simulink library "LIB_TF_G_12_StepControl"  (Simulink 8.6)
settings: Solver=ode45  StartTime=0.0  StopTime=10.0  RelTol=1e-3
PreLoadFcn:
  | if exist('tl_preloadfcn','file'), tl_preloadfcn(gcs,402); end
PostLoadFcn:
  | if exist('tl_postloadfcn','file'), tl_postloadfcn(gcs,402); end
undefined symbols (not defined in the file): ddv, u2, u3
libraries: tllib x4, LIB_TF_G_12_StepControl x1
(part 1 of 7)
CloseFcn:
  | if exist('tl_closefcn','file'), tl_closefcn(gcs); end
settings Model: TLRevision=402  Creator=cedric.sauvage  LastModifiedBy=audrey.vache

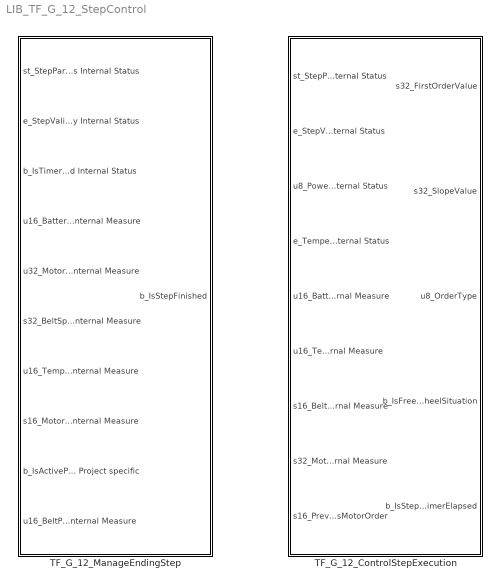
== system LIB_TF_G_12_StepControl ==
  TF_G_12_ControlStepExecution : Subsystem  TreatAsAtomicUnit=on
  TF_G_12_ManageEndingStep : Subsystem  TreatAsAtomicUnit=on

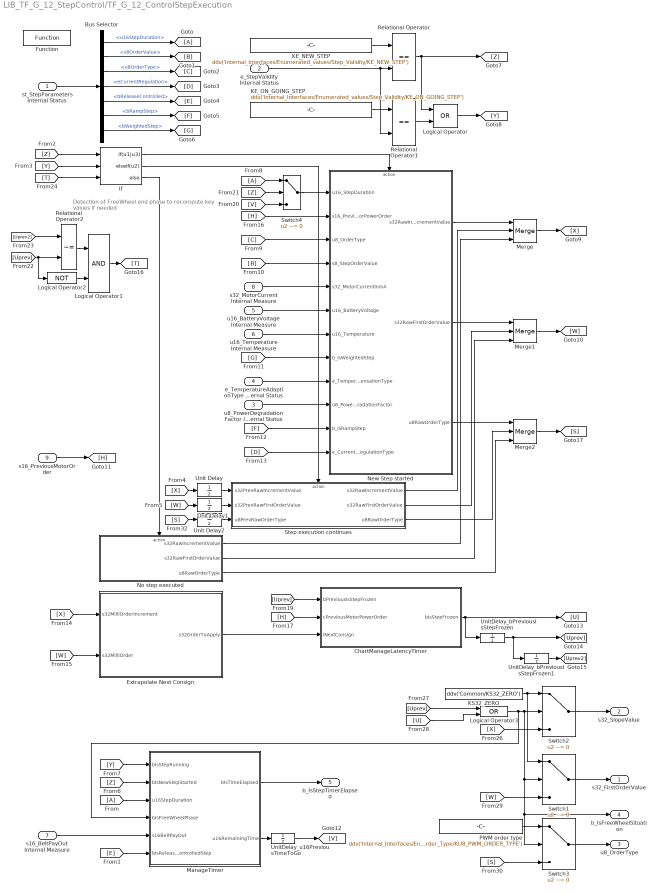
== system LIB_TF_G_12_StepControl/TF_G_12_ControlStepExecution ==
  note: Detection of FreeWheel end phase to recompute
      | key values if needed
  st_StepParameters Internal Status : Inport  OutDataTypeStr=Bus: stStepParameters
  e_StepValidity Internal Status : Inport  Port=2
  u8_PowerDegradationFactor Internal Status : Inport  Port=3
  e_TemperatureAdaptionType Internal Status : Inport  Port=4
  u16_BatteryVoltage Internal Measure : Inport  Port=5
  u16_Temperature Internal Measure : Inport  Port=6
  s16_BeltPayOut Internal Measure : Inport  Port=7
  s32_MotorCurrent Internal Measure : Inport  Port=8
  s16_PreviousMotorOrder : Inport  Port=9
  Bus Selector : BusSelector  OutputSignals=u16StepDuration,s8OrderValue,u8OrderType,eCurrentRegulation,bReleaseControlled,bRampStep,bWeightedStep
  ChartManageLatencyTimer : Stateflow chart  RequirementInfo={} %GIDa_4b5a57f6_b7b0_49a6_a1eb_944317c1d2de  TreatAsAtomicUnit=on
  Extrapolate Next Consign : Subsystem  RequirementInfo={} %GIDa_72e94147_9b66_478c_94cc_c32d89e0e2b0  TreatAsAtomicUnit=on
  Function : tllib/Function  RequirementInfo={'other' '..\..\..\..\Documents and Settings\cedric.sauvage\Desktop\BFE_Design.doc' '@Simulink_requirement_item_16' 'true' 'DSG_BFE_00033' '' } %GIDa_aa7399e7_4aec_40ce_b84e_da620cbb38ff  data={'stepfunctionname','M_ControlStepExecution','stepfunctionclass','STATIC_FCN_ASR4','codecomment',['[COVERS: DSG_BFE_00033]'],'date',736467.70154953701}  displayString=FUNCTION
  If : If  RequirementInfo={} %GIDa_dfdbd0a4_334d_4bd1_9cca_3fcb5b10a1a1  NumInputs=3  IfExpression=u1|u3  ElseIfExpressions=u2
  KE_NEW_STEP : Constant  Value=ddv('Internal_Interfaces/Enumerated_values/Step_Validity/KE_NEW_STEP')  mask(TL_Constant){data={'output',{'variable','Internal_Interfaces/Enumerated_values/Step_Validity/KE_NEW_STEP'},'date',735951.6680056944}}
      settings: CopyFcn=if exist('tl_reset_reviewflag','file')==2,tl_reset_reviewflag(gcbh);end  DeleteFcn=if exist('delete_tlblock','file')==2,delete_tlblock(gcbh);end  NameChangeFcn=if exist('rename_tlblock','file')==2,rename_tlblock(gcbh);end  OpenFcn=if exist('tl_open_blockdlg','file')==2,tl_open_blockdlg(gcbh);else,open_system(gcbh,'parameter');end
      mask Help: eval(['if exist(''tl_online_help'',''file'') == 2, tl_online_help(''Topic'',''TL_Constant''),else, web([''jar:file:///'',matlabroot,''/help/toolbox/simulink/help.jar!/slref/' lower(get_param(gcbh,'Blocktype')) '.html''], ''-helpbrowser''),end'])
      mask Display: plot([-0.05, 1.05, NaN, -0.05, 1.05],[.01, .01, NaN, .99, .99])
  KE_ON_GOING_STEP : Constant  Value=ddv('Internal_Interfaces/Enumerated_values/Step_Validity/KE_ON_GOING_STEP')  mask(TL_Constant){data={'output',{'variable','Internal_Interfaces/Enumerated_values/Step_Validity/KE_ON_GOING_STEP'},'date',735951.66800531244}}
      settings: CopyFcn=if exist('tl_reset_reviewflag','file')==2,tl_reset_reviewflag(gcbh);end  DeleteFcn=if exist('delete_tlblock','file')==2,delete_tlblock(gcbh);end  NameChangeFcn=if exist('rename_tlblock','file')==2,rename_tlblock(gcbh);end  OpenFcn=if exist('tl_open_blockdlg','file')==2,tl_open_blockdlg(gcbh);else,open_system(gcbh,'parameter');end
      mask Help: eval(['if exist(''tl_online_help'',''file'') == 2, tl_online_help(''Topic'',''TL_Constant''),else, web([''jar:file:///'',matlabroot,''/help/toolbox/simulink/help.jar!/slref/' lower(get_param(gcbh,'Blocktype')) '.html''], ''-helpbrowser''),end'])
      mask Display: plot([-0.05, 1.05, NaN, -0.05, 1.05],[.01, .01, NaN, .99, .99])
  KS32_ZERO : Constant  RequirementInfo={} %GIDa_9199cee5_bc37_4797_a880_19721e26adfa  Value=ddv('Common/KS32_ZERO')  OutDataTypeStr=int32  mask(TL_Constant){data={'output',{'variable','Common/KS32_ZERO'},'date',735951.66800494213}}
      settings: CopyFcn=if exist('tl_reset_reviewflag','file')==2,tl_reset_reviewflag(gcbh);end  DeleteFcn=if exist('delete_tlblock','file')==2,delete_tlblock(gcbh);end  NameChangeFcn=if exist('rename_tlblock','file')==2,rename_tlblock(gcbh);end  OpenFcn=if exist('tl_open_blockdlg','file')==2,tl_open_blockdlg(gcbh);else,open_system(gcbh,'parameter');end
      mask Help: eval(['if exist(''tl_online_help'',''file'') == 2, tl_online_help(''Topic'',''TL_Constant''),else, web([''jar:file:///'',matlabroot,''/help/toolbox/simulink/help.jar!/slref/' lower(get_param(gcbh,'Blocktype')) '.html''], ''-helpbrowser''),end'])
      mask Display: plot([-0.05, 1.05, NaN, -0.05, 1.05],[.01, .01, NaN, .99, .99])
  Logical Operator : Logic  Operator=OR  AllPortsSameDT=off  OutDataTypeStr=boolean  mask(TL_LogicalOperator){data={'output',{'name','bIsActiveStep'},'date',735951.66800458333}}
      settings: DeleteFcn=if exist('delete_tlblock','file')==2,delete_tlblock(gcbh);end  NameChangeFcn=if exist('rename_tlblock','file')==2,rename_tlblock(gcbh);end  OpenFcn=if exist('tl_open_blockdlg','file')==2,tl_open_blockdlg(gcbh);else,open_system(gcbh,'parameter');end
      mask Help: eval(['if exist(''tl_online_help'',''file'') == 2, tl_online_help(''Topic'',''TL_LogicalOperator''),else, web([''jar:file:///'',matlabroot,''/help/toolbox/simulink/help.jar!/slref/' lower(get_param(gcbh,'Blocktype')) '.html''], ''-helpbrowser''),end'])
      mask Display: plot([-0.05, 1.05, NaN, -0.05, 1.05],[.01, .01, NaN, .99, .99])
  Logical Operator1 : Logic  AllPortsSameDT=off  OutDataTypeStr=boolean  mask(TL_LogicalOperator){data={'output',{'name','bExitingFrozenState'},'date',735951.66800432873}}
      settings: DeleteFcn=if exist('delete_tlblock','file')==2,delete_tlblock(gcbh);end  NameChangeFcn=if exist('rename_tlblock','file')==2,rename_tlblock(gcbh);end  OpenFcn=if exist('tl_open_blockdlg','file')==2,tl_open_blockdlg(gcbh);else,open_system(gcbh,'parameter');end
      mask Help: eval(['if exist(''tl_online_help'',''file'') == 2, tl_online_help(''Topic'',''TL_LogicalOperator''),else, web([''jar:file:///'',matlabroot,''/help/toolbox/simulink/help.jar!/slref/' lower(get_param(gcbh,'Blocktype')) '.html''], ''-helpbrowser''),end'])
      mask Display: plot([-0.05, 1.05, NaN, -0.05, 1.05],[.01, .01, NaN, .99, .99])
  Logical Operator2 : Logic  Operator=NOT  Inputs=1  AllPortsSameDT=off  OutDataTypeStr=boolean  mask(TL_LogicalOperator){data={'date',735951.66800407402}}
      settings: DeleteFcn=if exist('delete_tlblock','file')==2,delete_tlblock(gcbh);end  NameChangeFcn=if exist('rename_tlblock','file')==2,rename_tlblock(gcbh);end  OpenFcn=if exist('tl_open_blockdlg','file')==2,tl_open_blockdlg(gcbh);else,open_system(gcbh,'parameter');end
      mask Help: eval(['if exist(''tl_online_help'',''file'') == 2, tl_online_help(''Topic'',''TL_LogicalOperator''),else, web([''jar:file:///'',matlabroot,''/help/toolbox/simulink/help.jar!/slref/' lower(get_param(gcbh,'Blocktype')) '.html''], ''-helpbrowser''),end'])
      mask Display: plot([-0.05, 1.05, NaN, -0.05, 1.05],[.01, .01, NaN, .99, .99])
  Logical Operator3 : Logic  Operator=OR  AllPortsSameDT=off  OutDataTypeStr=boolean  mask(TL_LogicalOperator){data={'output',{'name','bIsFreeWheelingState'},'date',735951.66800378473}}
      settings: DeleteFcn=if exist('delete_tlblock','file')==2,delete_tlblock(gcbh);end  NameChangeFcn=if exist('rename_tlblock','file')==2,rename_tlblock(gcbh);end  OpenFcn=if exist('tl_open_blockdlg','file')==2,tl_open_blockdlg(gcbh);else,open_system(gcbh,'parameter');end
      mask Help: eval(['if exist(''tl_online_help'',''file'') == 2, tl_online_help(''Topic'',''TL_LogicalOperator''),else, web([''jar:file:///'',matlabroot,''/help/toolbox/simulink/help.jar!/slref/' lower(get_param(gcbh,'Blocktype')) '.html''], ''-helpbrowser''),end'])
      mask Display: plot([-0.05, 1.05, NaN, -0.05, 1.05],[.01, .01, NaN, .99, .99])
  ManageTimer : Subsystem  RequirementInfo={} %GIDa_1c6e116c_deb6_4c8b_9c2a_a3ed8f535171  TreatAsAtomicUnit=on
      settings: RTWFcnNameOpts=Use subsystem name
  Merge : Merge  Inputs=3  InitialOutput=0  mask(TL_Merge){data={'output',{'name','s32RawIncrementValue'},'date',735951.66799646989}}
      settings: CopyFcn=if exist('tl_reset_reviewflag','file')==2,tl_reset_reviewflag(gcbh);end  DeleteFcn=if exist('delete_tlblock','file')==2,delete_tlblock(gcbh);end  NameChangeFcn=if exist('rename_tlblock','file')==2,rename_tlblock(gcbh);end  OpenFcn=if exist('tl_open_blockdlg','file')==2,tl_open_blockdlg(gcbh);else,open_system(gcbh,'parameter');end
      mask Help: eval(['if exist(''tl_online_help'',''file'') == 2, tl_online_help(''Topic'',''TL_Merge''),else, web([''jar:file:///'',matlabroot,''/help/toolbox/simulink/help.jar!/slref/' lower(get_param(gcbh,'Blocktype')) '.html''], ''-helpbrowser''),end'])
      mask Display: plot([-0.05, 1.05, NaN, -0.05, 1.05],[.01, .01, NaN, .99, .99])
  Merge1 : Merge  Inputs=3  InitialOutput=0  mask(TL_Merge){data={'output',{'name','s32RawFirstOrderValue'},'date',735951.66799608793}}
      settings: CopyFcn=if exist('tl_reset_reviewflag','file')==2,tl_reset_reviewflag(gcbh);end  DeleteFcn=if exist('delete_tlblock','file')==2,delete_tlblock(gcbh);end  NameChangeFcn=if exist('rename_tlblock','file')==2,rename_tlblock(gcbh);end  OpenFcn=if exist('tl_open_blockdlg','file')==2,tl_open_blockdlg(gcbh);else,open_system(gcbh,'parameter');end
      mask Help: eval(['if exist(''tl_online_help'',''file'') == 2, tl_online_help(''Topic'',''TL_Merge''),else, web([''jar:file:///'',matlabroot,''/help/toolbox/simulink/help.jar!/slref/' lower(get_param(gcbh,'Blocktype')) '.html''], ''-helpbrowser''),end'])
      mask Display: plot([-0.05, 1.05, NaN, -0.05, 1.05],[.01, .01, NaN, .99, .99])
  Merge2 : Merge  RequirementInfo={} %GIDa_81538ec5_5da8_4e36_98a9_b64854f730e2  Inputs=3  InitialOutput=0  mask(TL_Merge){data={'output',{'name','u8RawOrderType'},'date',735951.66799569444}}
      settings: CopyFcn=if exist('tl_reset_reviewflag','file')==2,tl_reset_reviewflag(gcbh);end  DeleteFcn=if exist('delete_tlblock','file')==2,delete_tlblock(gcbh);end  NameChangeFcn=if exist('rename_tlblock','file')==2,rename_tlblock(gcbh);end  OpenFcn=if exist('tl_open_blockdlg','file')==2,tl_open_blockdlg(gcbh);else,open_system(gcbh,'parameter');end
      mask Help: eval(['if exist(''tl_online_help'',''file'') == 2, tl_online_help(''Topic'',''TL_Merge''),else, web([''jar:file:///'',matlabroot,''/help/toolbox/simulink/help.jar!/slref/' lower(get_param(gcbh,'Blocktype')) '.html''], ''-helpbrowser''),end'])
      mask Display: plot([-0.05, 1.05, NaN, -0.05, 1.05],[.01, .01, NaN, .99, .99])
  New Step started : Subsystem  TreatAsAtomicUnit=on
  No step executed : Subsystem  TreatAsAtomicUnit=on
  PWM order type : Constant  Value=ddv('Internal_Interfaces/Enumerated_values/Step_Order_Type/KU8_PWM_ORDER_TYPE')  OutDataTypeStr=uint8  mask(TL_Constant){data={'output',{'variable','Internal_Interfaces/Enumerated_values/Step_Order_Type/KU8_PWM_ORDER_TYPE'},'date',735951.66796200234}}
      settings: CopyFcn=if exist('tl_reset_reviewflag','file')==2,tl_reset_reviewflag(gcbh);end  DeleteFcn=if exist('delete_tlblock','file')==2,delete_tlblock(gcbh);end  NameChangeFcn=if exist('rename_tlblock','file')==2,rename_tlblock(gcbh);end  OpenFcn=if exist('tl_open_blockdlg','file')==2,tl_open_blockdlg(gcbh);else,open_system(gcbh,'parameter');end
      mask Help: eval(['if exist(''tl_online_help'',''file'') == 2, tl_online_help(''Topic'',''TL_Constant''),else, web([''jar:file:///'',matlabroot,''/help/toolbox/simulink/help.jar!/slref/' lower(get_param(gcbh,'Blocktype')) '.html''], ''-helpbrowser''),end'])
      mask Display: plot([-0.05, 1.05, NaN, -0.05, 1.05],[.01, .01, NaN, .99, .99])
  Relational Operator : RelationalOperator  Operator===  OutDataTypeStr=boolean  mask(TL_RelationalOperator){data={'output',{'name','bIsNewStepStarted'},'date',735951.66796164354}}
      settings: DeleteFcn=if exist('delete_tlblock','file')==2,delete_tlblock(gcbh);end  NameChangeFcn=if exist('rename_tlblock','file')==2,rename_tlblock(gcbh);end  OpenFcn=if exist('tl_open_blockdlg','file')==2,tl_open_blockdlg(gcbh);else,open_system(gcbh,'parameter');end
      mask Help: eval(['if exist(''tl_online_help'',''file'') == 2, tl_online_help(''Topic'',''TL_RelationalOperator''),else, web([''jar:file:///'',matlabroot,''/help/toolbox/simulink/help.jar!/slref/' lower(get_param(gcbh,'Blocktype')) '.html''], ''-helpbrowser''),end'])
      mask Display: plot([-0.05, 1.05, NaN, -0.05, 1.05],[.01, .01, NaN, .99, .99])
  Relational Operator1 : RelationalOperator  Operator===  OutDataTypeStr=boolean  mask(TL_RelationalOperator){data={'date',735951.66796138894}}
      settings: DeleteFcn=if exist('delete_tlblock','file')==2,delete_tlblock(gcbh);end  NameChangeFcn=if exist('rename_tlblock','file')==2,rename_tlblock(gcbh);end  OpenFcn=if exist('tl_open_blockdlg','file')==2,tl_open_blockdlg(gcbh);else,open_system(gcbh,'parameter');end
      mask Help: eval(['if exist(''tl_online_help'',''file'') == 2, tl_online_help(''Topic'',''TL_RelationalOperator''),else, web([''jar:file:///'',matlabroot,''/help/toolbox/simulink/help.jar!/slref/' lower(get_param(gcbh,'Blocktype')) '.html''], ''-helpbrowser''),end'])
      mask Display: plot([-0.05, 1.05, NaN, -0.05, 1.05],[.01, .01, NaN, .99, .99])
  Relational Operator2 : RelationalOperator  Operator=~=  OutDataTypeStr=boolean  mask(TL_RelationalOperator){data={'date',735951.66796114587}}
      settings: DeleteFcn=if exist('delete_tlblock','file')==2,delete_tlblock(gcbh);end  NameChangeFcn=if exist('rename_tlblock','file')==2,rename_tlblock(gcbh);end  OpenFcn=if exist('tl_open_blockdlg','file')==2,tl_open_blockdlg(gcbh);else,open_system(gcbh,'parameter');end
      mask Help: eval(['if exist(''tl_online_help'',''file'') == 2, tl_online_help(''Topic'',''TL_RelationalOperator''),else, web([''jar:file:///'',matlabroot,''/help/toolbox/simulink/help.jar!/slref/' lower(get_param(gcbh,'Blocktype')) '.html''], ''-helpbrowser''),end'])
      mask Display: plot([-0.05, 1.05, NaN, -0.05, 1.05],[.01, .01, NaN, .99, .99])
  Step execution continues : Subsystem  TreatAsAtomicUnit=on
  Switch1 : Switch  RequirementInfo={} %GIDa_65f15ba1_d201_44dd_96e9_da7c8589fb96  Criteria=u2 ~= 0  mask(TL_Switch){data={'output',{'name','s32FirstOrderFiltered','type','Int32'},'threshold',{'scalar',1},'date',735951.66796084493}}
      settings: CopyFcn=if exist('tl_reset_reviewflag','file')==2,tl_reset_reviewflag(gcbh);end  DeleteFcn=if exist('delete_tlblock','file')==2,delete_tlblock(gcbh);end  NameChangeFcn=if exist('rename_tlblock','file')==2,rename_tlblock(gcbh);end  OpenFcn=if exist('tl_open_blockdlg','file')==2,tl_open_blockdlg(gcbh);else,open_system(gcbh,'parameter');end
      mask Help: eval(['if exist(''tl_online_help'',''file'') == 2, tl_online_help(''Topic'',''TL_Switch''),else, web([''jar:file:///'',matlabroot,''/help/toolbox/simulink/help.jar!/slref/' lower(get_param(gcbh,'Blocktype')) '.html''], ''-helpbrowser''),end'])
      mask Display: plot([-0.05, 1.05, NaN, -0.05, 1.05],[.01, .01, NaN, .99, .99])
  Switch2 : Switch  RequirementInfo={} %GIDa_a7c51ab5_8b03_4252_98c7_56702c939012  Criteria=u2 ~= 0  mask(TL_Switch){data={'output',{'name','s32IncrementFiltered','type','Int32'},'date',735951.66796031245}}
      settings: CopyFcn=if exist('tl_reset_reviewflag','file')==2,tl_reset_reviewflag(gcbh);end  DeleteFcn=if exist('delete_tlblock','file')==2,delete_tlblock(gcbh);end  NameChangeFcn=if exist('rename_tlblock','file')==2,rename_tlblock(gcbh);end  OpenFcn=if exist('tl_open_blockdlg','file')==2,tl_open_blockdlg(gcbh);else,open_system(gcbh,'parameter');end
      mask Help: eval(['if exist(''tl_online_help'',''file'') == 2, tl_online_help(''Topic'',''TL_Switch''),else, web([''jar:file:///'',matlabroot,''/help/toolbox/simulink/help.jar!/slref/' lower(get_param(gcbh,'Blocktype')) '.html''], ''-helpbrowser''),end'])
      mask Display: plot([-0.05, 1.05, NaN, -0.05, 1.05],[.01, .01, NaN, .99, .99])
  Switch3 : Switch  RequirementInfo={} %GIDa_04cbf39d_4ae3_4f39_b284_4319f63f0cce  Criteria=u2 ~= 0  mask(TL_Switch){data={'output',{'name','u8OrderTypeFiltered','type','UInt8'},'date',735951.66795978008}}
      settings: CopyFcn=if exist('tl_reset_reviewflag','file')==2,tl_reset_reviewflag(gcbh);end  DeleteFcn=if exist('delete_tlblock','file')==2,delete_tlblock(gcbh);end  NameChangeFcn=if exist('rename_tlblock','file')==2,rename_tlblock(gcbh);end  OpenFcn=if exist('tl_open_blockdlg','file')==2,tl_open_blockdlg(gcbh);else,open_system(gcbh,'parameter');end
      mask Help: eval(['if exist(''tl_online_help'',''file'') == 2, tl_online_help(''Topic'',''TL_Switch''),else, web([''jar:file:///'',matlabroot,''/help/toolbox/simulink/help.jar!/slref/' lower(get_param(gcbh,'Blocktype')) '.html''], ''-helpbrowser''),end'])
      mask Display: plot([-0.05, 1.05, NaN, -0.05, 1.05],[.01, .01, NaN, .99, .99])
  Switch4 : Switch  RequirementInfo={} %GIDa_6dc782cd_9c7f_43a9_a347_f998369ad35f  Criteria=u2 ~= 0  mask(TL_Switch){data={'output',{'inheritscaling',1},'threshold',{'scalar',1},'date',735951.66795924772}}
      settings: CopyFcn=if exist('tl_reset_reviewflag','file')==2,tl_reset_reviewflag(gcbh);end  DeleteFcn=if exist('delete_tlblock','file')==2,delete_tlblock(gcbh);end  NameChangeFcn=if exist('rename_tlblock','file')==2,rename_tlblock(gcbh);end  OpenFcn=if exist('tl_open_blockdlg','file')==2,tl_open_blockdlg(gcbh);else,open_system(gcbh,'parameter');end
      mask Help: eval(['if exist(''tl_online_help'',''file'') == 2, tl_online_help(''Topic'',''TL_Switch''),else, web([''jar:file:///'',matlabroot,''/help/toolbox/simulink/help.jar!/slref/' lower(get_param(gcbh,'Blocktype')) '.html''], ''-helpbrowser''),end'])
      mask Display: plot([-0.05, 1.05, NaN, -0.05, 1.05],[.01, .01, NaN, .99, .99])
  Unit Delay : UnitDelay  SampleTime=-1  mask(TL_UnitDelay){data={'output',{'type','Int32'},'state',{'name','s32PrevRawIncrementValue','type','Int32'},'date',735951.66795871523}}
      settings: CopyFcn=if exist('tl_reset_reviewflag','file')==2,tl_reset_reviewflag(gcbh);end  DeleteFcn=if exist('delete_tlblock','file')==2,delete_tlblock(gcbh);end  NameChangeFcn=if exist('rename_tlblock','file')==2,rename_tlblock(gcbh);end  OpenFcn=if exist('tl_open_blockdlg','file')==2,tl_open_blockdlg(gcbh);else,open_system(gcbh,'parameter');end
      mask Help: eval(['if exist(''tl_online_help'',''file'') == 2, tl_online_help(''Topic'',''TL_UnitDelay''),else, web([''jar:file:///'',matlabroot,''/help/toolbox/simulink/help.jar!/slref/' lower(get_param(gcbh,'Blocktype')) '.html''], ''-helpbrowser''),end'])
      mask Display: plot([-0.05, 1.05, NaN, -0.05, 1.05],[.01, .01, NaN, .99, .99])
  Unit Delay1 : UnitDelay  SampleTime=-1  mask(TL_UnitDelay){data={'output',{'type','Int32'},'state',{'name','s32PrevRawFirstOrderValue','type','Int32'},'date',735951.66795818286}}
      settings: CopyFcn=if exist('tl_reset_reviewflag','file')==2,tl_reset_reviewflag(gcbh);end  DeleteFcn=if exist('delete_tlblock','file')==2,delete_tlblock(gcbh);end  NameChangeFcn=if exist('rename_tlblock','file')==2,rename_tlblock(gcbh);end  OpenFcn=if exist('tl_open_blockdlg','file')==2,tl_open_blockdlg(gcbh);else,open_system(gcbh,'parameter');end
      mask Help: eval(['if exist(''tl_online_help'',''file'') == 2, tl_online_help(''Topic'',''TL_UnitDelay''),else, web([''jar:file:///'',matlabroot,''/help/toolbox/simulink/help.jar!/slref/' lower(get_param(gcbh,'Blocktype')) '.html''], ''-helpbrowser''),end'])
      mask Display: plot([-0.05, 1.05, NaN, -0.05, 1.05],[.01, .01, NaN, .99, .99])
  Unit Delay2 : UnitDelay  SampleTime=-1  mask(TL_UnitDelay){data={'output',{'type','UInt8'},'state',{'name','u8PrevRawOrderType','type','UInt8'},'date',735951.66795767366}}
      settings: CopyFcn=if exist('tl_reset_reviewflag','file')==2,tl_reset_reviewflag(gcbh);end  DeleteFcn=if exist('delete_tlblock','file')==2,delete_tlblock(gcbh);end  NameChangeFcn=if exist('rename_tlblock','file')==2,rename_tlblock(gcbh);end  OpenFcn=if exist('tl_open_blockdlg','file')==2,tl_open_blockdlg(gcbh);else,open_system(gcbh,'parameter');end
      mask Help: eval(['if exist(''tl_online_help'',''file'') == 2, tl_online_help(''Topic'',''TL_UnitDelay''),else, web([''jar:file:///'',matlabroot,''/help/toolbox/simulink/help.jar!/slref/' lower(get_param(gcbh,'Blocktype')) '.html''], ''-helpbrowser''),end'])
      mask Display: plot([-0.05, 1.05, NaN, -0.05, 1.05],[.01, .01, NaN, .99, .99])
  UnitDelay_bPreviousIsStepFrozen : UnitDelay  RequirementInfo={} %GIDa_488b8b5e_6cfd_47d8_a17a_2b83159a3d65  SampleTime=-1  mask(TL_UnitDelay){data={'output',{'type','Bool'},'state',{'name','bOldFrozenStep','type','Bool'},'date',735951.66795716435}}
      settings: CopyFcn=if exist('tl_reset_reviewflag','file')==2,tl_reset_reviewflag(gcbh);end  DeleteFcn=if exist('delete_tlblock','file')==2,delete_tlblock(gcbh);end  NameChangeFcn=if exist('rename_tlblock','file')==2,rename_tlblock(gcbh);end  OpenFcn=if exist('tl_open_blockdlg','file')==2,tl_open_blockdlg(gcbh);else,open_system(gcbh,'parameter');end
      mask Help: eval(['if exist(''tl_online_help'',''file'') == 2, tl_online_help(''Topic'',''TL_UnitDelay''),else, web([''jar:file:///'',matlabroot,''/help/toolbox/simulink/help.jar!/slref/' lower(get_param(gcbh,'Blocktype')) '.html''], ''-helpbrowser''),end'])
      mask Display: plot([-0.05, 1.05, NaN, -0.05, 1.05],[.01, .01, NaN, .99, .99])
  UnitDelay_bPreviousIsStepFrozen1 : UnitDelay  RequirementInfo={} %GIDa_66da4426_fc4d_4144_a53c_1e2d3e1577c6  SampleTime=-1  mask(TL_UnitDelay){data={'output',{'type','Bool'},'state',{'name','bOldFrozenStep2','type','Bool'},'date',735951.66795664351}}
      settings: CopyFcn=if exist('tl_reset_reviewflag','file')==2,tl_reset_reviewflag(gcbh);end  DeleteFcn=if exist('delete_tlblock','file')==2,delete_tlblock(gcbh);end  NameChangeFcn=if exist('rename_tlblock','file')==2,rename_tlblock(gcbh);end  OpenFcn=if exist('tl_open_blockdlg','file')==2,tl_open_blockdlg(gcbh);else,open_system(gcbh,'parameter');end
      mask Help: eval(['if exist(''tl_online_help'',''file'') == 2, tl_online_help(''Topic'',''TL_UnitDelay''),else, web([''jar:file:///'',matlabroot,''/help/toolbox/simulink/help.jar!/slref/' lower(get_param(gcbh,'Blocktype')) '.html''], ''-helpbrowser''),end'])
      mask Display: plot([-0.05, 1.05, NaN, -0.05, 1.05],[.01, .01, NaN, .99, .99])
  UnitDelay_u16PreviousTimeToGo : UnitDelay  RequirementInfo={} %GIDa_419bb3ad_f2bc_43ef_96dd_121e9a048b47  SampleTime=-1  mask(TL_UnitDelay){data={'output',{'type','UInt16'},'state',{'name','u16PrevRemainingTime','type','UInt16'},'date',735951.6679561343}}
      settings: CopyFcn=if exist('tl_reset_reviewflag','file')==2,tl_reset_reviewflag(gcbh);end  DeleteFcn=if exist('delete_tlblock','file')==2,delete_tlblock(gcbh);end  NameChangeFcn=if exist('rename_tlblock','file')==2,rename_tlblock(gcbh);end  OpenFcn=if exist('tl_open_blockdlg','file')==2,tl_open_blockdlg(gcbh);else,open_system(gcbh,'parameter');end
      mask Help: eval(['if exist(''tl_online_help'',''file'') == 2, tl_online_help(''Topic'',''TL_UnitDelay''),else, web([''jar:file:///'',matlabroot,''/help/toolbox/simulink/help.jar!/slref/' lower(get_param(gcbh,'Blocktype')) '.html''], ''-helpbrowser''),end'])
      mask Display: plot([-0.05, 1.05, NaN, -0.05, 1.05],[.01, .01, NaN, .99, .99])
  s32_FirstOrderValue : Outport
  s32_SlopeValue : Outport  Port=2
  u8_OrderType : Outport  Port=3
  b_IsFreeWheelSituation : Outport  Port=4
  b_IsStepTimerElapsed : Outport  Port=5
  wires:
  [S] -> Switch3/3
  [S] -> Unit Delay2/1
  Merge2/1 -> [S]
  No step executed/3(u8RawOrderType) -> Merge2/3
  Step execution continues/3(u8RawOrderType) -> Merge2/2
  New Step started/3(u8RawOrderType) -> Merge2/1
  Unit Delay2/1 -> Step execution continues/3(u8PrevRawOrderType)
  st_StepParameters Internal Status/1 -> Bus Selector/1
  Bus Selector/1 -> [A]  "<u16StepDuration>"
  Bus Selector/2 -> [B]  "<s8OrderValue>"
  Bus Selector/3 -> [C]  "<u8OrderType>"
  Bus Selector/4 -> [D]  "<eCurrentRegulation>"
  Bus Selector/5 -> [E]  "<bReleaseControlled>"
  Bus Selector/6 -> [F]  "<bRampStep>"
  Bus Selector/7 -> [G]  "<bWeightedStep>"
  ManageTimer/1(bIsTimeElapsed) -> b_IsStepTimerElapsed/1
  [A] -> ManageTimer/3(u16StepDuration)
  [E] -> ManageTimer/6(bIsReleasedControlledStep)
  s16_BeltPayOut Internal Measure/1 -> ManageTimer/5(s16BeltPayOut)
  e_StepValidity Internal Status/1 -> Relational Operator/2, Relational Operator1/2
  KE_NEW_STEP/1 -> Relational Operator/1
  KE_ON_GOING_STEP/1 -> Relational Operator1/1
  Relational Operator1/1 -> Logical Operator/2
  Relational Operator/1 -> Logical Operator/1, [Z]
  Logical Operator/1 -> [Y]
  [Z] -> If/1
  If/1 -> New Step started/Action
  [Y] -> If/2
  If/2 -> Step execution continues/Action
  If/3 -> No step executed/Action
  New Step started/1(s32RawIncrementValue) -> Merge/1
  New Step started/2(s32RawFirstOrderValue) -> Merge1/1
  Step execution continues/1(s32RawIncrementValue) -> Merge/2
  No step executed/1(s32RawIncrementValue) -> Merge/3
  Step execution continues/2(s32RawFirstOrderValue) -> Merge1/2
  No step executed/2(s32RawFirstOrderValue) -> Merge1/3
  [X] -> Unit Delay/1
  Unit Delay/1 -> Step execution continues/1(s32PrevRawIncrementValue)
  [W] -> Unit Delay1/1
  Unit Delay1/1 -> Step execution continues/2(s32PrevRawFirstOrderValue)
  Merge/1 -> [X]
  Merge1/1 -> [W]
  [Z] -> ManageTimer/2(bIsNewStepStarted)
  [Y] -> ManageTimer/1(bIsStepRunning)
  u8_PowerDegradationFactor Internal Status/1 -> New Step started/10(u8_PowerDegradationFactor)
  e_TemperatureAdaptionType Internal Status/1 -> New Step started/9(e_TemperatureCompensationType)
  u16_BatteryVoltage Internal Measure/1 -> New Step started/6(u16_BatteryVoltage)
  u16_Temperature Internal Measure/1 -> New Step started/7(u16_Temperature)
  s32_MotorCurrent Internal Measure/1 -> New Step started/5(s32_MotorCurrentInmA)
  Switch4/1 -> New Step started/1(u16_StepDuration)
  [C] -> New Step started/3(u8_OrderType)
  [B] -> New Step started/4(s8_StepOrderValue)
  [G] -> New Step started/8(b_IsWeightedStep)
  [F] -> New Step started/11(b_IsRampStep)
  [D] -> New Step started/12(e_CurrentRegulationType)
  [W] -> Extrapolate Next Consign/2(s32MilliOrder)
  [X] -> Extrapolate Next Consign/1(s32MilliOrderIncrement)
  ManageTimer/2(u16RemainingTime) -> UnitDelay_u16PreviousTimeToGo/1
  [H] -> New Step started/2(s16_PreviousMotorPowerOrder)
  s16_PreviousMotorOrder/1 -> [H]
  [H] -> ChartManageLatencyTimer/2(cPreviousMotorPowerOrder)
  UnitDelay_u16PreviousTimeToGo/1 -> [V]
  Extrapolate Next Consign/1(s32OrderToApply) -> ChartManageLatencyTimer/3(lNextConsign)
  ChartManageLatencyTimer/1(bIsStepFrozen) -> UnitDelay_bPreviousIsStepFrozen/1, [U]
  UnitDelay_bPreviousIsStepFrozen/1 -> [Uprev], UnitDelay_bPreviousIsStepFrozen1/1
  Logical Operator3/1 -> ManageTimer/4(bIsFreeWheelPhase), Switch2/2, b_IsFreeWheelSituation/1, Switch3/2, Switch1/2
  [Uprev] -> ChartManageLatencyTimer/1(bPreviousIsStepFrozen)
  [A] -> Switch4/1
  [V] -> Switch4/3
  [Z] -> Switch4/2
  UnitDelay_bPreviousIsStepFrozen1/1 -> [Uprev2]
  Relational Operator2/1 -> Logical Operator1/1
  [Uprev] -> Relational Operator2/2, Logical Operator2/1
  [Uprev2] -> Relational Operator2/1
  Logical Operator2/1 -> Logical Operator1/2
  Logical Operator1/1 -> [T]
  [T] -> If/3
  KS32_ZERO/1 -> Switch2/1, Switch1/1
  Switch2/1 -> s32_SlopeValue/1
  [X] -> Switch2/3
  [Uprev] -> Logical Operator3/1
  [U] -> Logical Operator3/2
  Switch1/1 -> s32_FirstOrderValue/1
  [W] -> Switch1/3
  Switch3/1 -> u8_OrderType/1
  PWM order type/1 -> Switch3/1

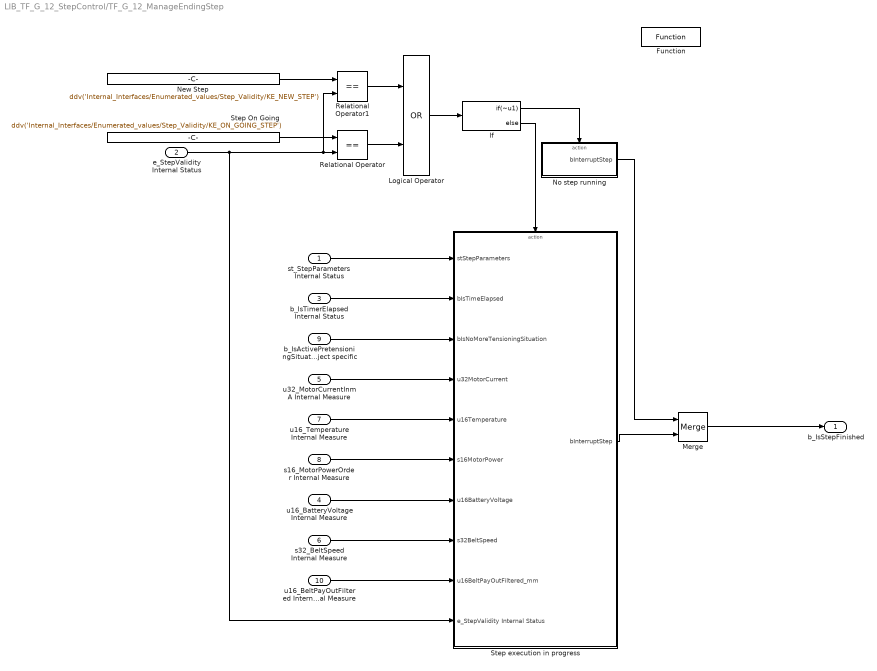
== system LIB_TF_G_12_StepControl/TF_G_12_ManageEndingStep ==
  st_StepParameters Internal Status : Inport  OutDataTypeStr=Bus: stStepParameters
  e_StepValidity Internal Status : Inport  Port=2
  b_IsTimerElapsed Internal Status : Inport  Port=3
  u16_BatteryVoltage Internal Measure : Inport  Port=4
  u32_MotorCurrentInmA Internal Measure : Inport  Port=5
  s32_BeltSpeed Internal Measure : Inport  Port=6
  u16_Temperature Internal Measure : Inport  Port=7
  s16_MotorPowerOrder Internal Measure : Inport  Port=8
  b_IsActivePretensioningSituation Project specific : Inport  Port=9
  u16_BeltPayOutFiltered Internal Measure : Inport  Port=10
  Function : tllib/Function  RequirementInfo={} %GIDa_9a6d8b05_ba8e_46f3_971b_8d797ff25032  data={'stepfunctionname','M_ManageStepEvents','stepfunctionclass','STATIC_FCN_ASR4','restartfunctionname','RESTART_ManageStepEvents','initfunctionname','INIT_ManageStepEvents','termfunctionname','TERM_ManageStepEvents','subsystemid','c','date',736467.70168917824}  displayString=FUNCTION
  If : If  RequirementInfo={} %GIDa_cfa7aa71_322d_4446_9931_a2ed9032b64a  IfExpression=~u1
  Logical Operator : Logic  Operator=OR  AllPortsSameDT=off  OutDataTypeStr=boolean  mask(TL_LogicalOperator){data={'output',{'name','bIsStepExecutionOnGoing'},'date',735951.66848681716}}
      settings: DeleteFcn=if exist('delete_tlblock','file')==2,delete_tlblock(gcbh);end  NameChangeFcn=if exist('rename_tlblock','file')==2,rename_tlblock(gcbh);end  OpenFcn=if exist('tl_open_blockdlg','file')==2,tl_open_blockdlg(gcbh);else,open_system(gcbh,'parameter');end
      mask Help: eval(['if exist(''tl_online_help'',''file'') == 2, tl_online_help(''Topic'',''TL_LogicalOperator''),else, web([''jar:file:///'',matlabroot,''/help/toolbox/simulink/help.jar!/slref/' lower(get_param(gcbh,'Blocktype')) '.html''], ''-helpbrowser''),end'])
      mask Display: plot([-0.05, 1.05, NaN, -0.05, 1.05],[.01, .01, NaN, .99, .99])
  Merge : Merge  RequirementInfo={} %GIDa_b284fdd1_e539_49dd_8c60_3fc7cb7526ed  InitialOutput=1  mask(TL_Merge){data={'output',{'name','bIsStepFinished'},'date',735951.66848655092}}
      settings: CopyFcn=if exist('tl_reset_reviewflag','file')==2,tl_reset_reviewflag(gcbh);end  DeleteFcn=if exist('delete_tlblock','file')==2,delete_tlblock(gcbh);end  NameChangeFcn=if exist('rename_tlblock','file')==2,rename_tlblock(gcbh);end  OpenFcn=if exist('tl_open_blockdlg','file')==2,tl_open_blockdlg(gcbh);else,open_system(gcbh,'parameter');end
      mask Help: eval(['if exist(''tl_online_help'',''file'') == 2, tl_online_help(''Topic'',''TL_Merge''),else, web([''jar:file:///'',matlabroot,''/help/toolbox/simulink/help.jar!/slref/' lower(get_param(gcbh,'Blocktype')) '.html''], ''-helpbrowser''),end'])
      mask Display: plot([-0.05, 1.05, NaN, -0.05, 1.05],[.01, .01, NaN, .99, .99])
  New Step : Constant  Value=ddv('Internal_Interfaces/Enumerated_values/Step_Validity/KE_NEW_STEP')  mask(TL_Constant){data={'output',{'variable','Internal_Interfaces/Enumerated_values/Step_Validity/KE_NEW_STEP'},'date',735951.6684861806}}
      settings: CopyFcn=if exist('tl_reset_reviewflag','file')==2,tl_reset_reviewflag(gcbh);end  DeleteFcn=if exist('delete_tlblock','file')==2,delete_tlblock(gcbh);end  NameChangeFcn=if exist('rename_tlblock','file')==2,rename_tlblock(gcbh);end  OpenFcn=if exist('tl_open_blockdlg','file')==2,tl_open_blockdlg(gcbh);else,open_system(gcbh,'parameter');end
      mask Help: eval(['if exist(''tl_online_help'',''file'') == 2, tl_online_help(''Topic'',''TL_Constant''),else, web([''jar:file:///'',matlabroot,''/help/toolbox/simulink/help.jar!/slref/' lower(get_param(gcbh,'Blocktype')) '.html''], ''-helpbrowser''),end'])
      mask Display: plot([-0.05, 1.05, NaN, -0.05, 1.05],[.01, .01, NaN, .99, .99])
  No step running : Subsystem  RequirementInfo={} %GIDa_99bb8b7e_6195_4028_afab_1d591910ff1a  TreatAsAtomicUnit=on
  Relational Operator : RelationalOperator  Operator===  OutDataTypeStr=boolean  mask(TL_RelationalOperator){data={'date',735951.66848545137}}
      settings: DeleteFcn=if exist('delete_tlblock','file')==2,delete_tlblock(gcbh);end  NameChangeFcn=if exist('rename_tlblock','file')==2,rename_tlblock(gcbh);end  OpenFcn=if exist('tl_open_blockdlg','file')==2,tl_open_blockdlg(gcbh);else,open_system(gcbh,'parameter');end
      mask Help: eval(['if exist(''tl_online_help'',''file'') == 2, tl_online_help(''Topic'',''TL_RelationalOperator''),else, web([''jar:file:///'',matlabroot,''/help/toolbox/simulink/help.jar!/slref/' lower(get_param(gcbh,'Blocktype')) '.html''], ''-helpbrowser''),end'])
      mask Display: plot([-0.05, 1.05, NaN, -0.05, 1.05],[.01, .01, NaN, .99, .99])
  Relational Operator1 : RelationalOperator  Operator===  OutDataTypeStr=boolean  mask(TL_RelationalOperator){data={'date',735951.6684852083}}
      settings: DeleteFcn=if exist('delete_tlblock','file')==2,delete_tlblock(gcbh);end  NameChangeFcn=if exist('rename_tlblock','file')==2,rename_tlblock(gcbh);end  OpenFcn=if exist('tl_open_blockdlg','file')==2,tl_open_blockdlg(gcbh);else,open_system(gcbh,'parameter');end
      mask Help: eval(['if exist(''tl_online_help'',''file'') == 2, tl_online_help(''Topic'',''TL_RelationalOperator''),else, web([''jar:file:///'',matlabroot,''/help/toolbox/simulink/help.jar!/slref/' lower(get_param(gcbh,'Blocktype')) '.html''], ''-helpbrowser''),end'])
      mask Display: plot([-0.05, 1.05, NaN, -0.05, 1.05],[.01, .01, NaN, .99, .99])
  Step On Going : Constant  Value=ddv('Internal_Interfaces/Enumerated_values/Step_Validity/KE_ON_GOING_STEP')  mask(TL_Constant){data={'output',{'variable','Internal_Interfaces/Enumerated_values/Step_Validity/KE_ON_GOING_STEP'},'date',735951.6684849537}}
      settings: CopyFcn=if exist('tl_reset_reviewflag','file')==2,tl_reset_reviewflag(gcbh);end  DeleteFcn=if exist('delete_tlblock','file')==2,delete_tlblock(gcbh);end  NameChangeFcn=if exist('rename_tlblock','file')==2,rename_tlblock(gcbh);end  OpenFcn=if exist('tl_open_blockdlg','file')==2,tl_open_blockdlg(gcbh);else,open_system(gcbh,'parameter');end
      mask Help: eval(['if exist(''tl_online_help'',''file'') == 2, tl_online_help(''Topic'',''TL_Constant''),else, web([''jar:file:///'',matlabroot,''/help/toolbox/simulink/help.jar!/slref/' lower(get_param(gcbh,'Blocktype')) '.html''], ''-helpbrowser''),end'])
      mask Display: plot([-0.05, 1.05, NaN, -0.05, 1.05],[.01, .01, NaN, .99, .99])
  Step execution in progress : Subsystem  RequirementInfo={} %GIDa_651d3e86_3fde_41a6_a5b3_45e8f0aed5c5  TreatAsAtomicUnit=on
  b_IsStepFinished : Outport
  wires:
  If/1 -> No step running/Action
  If/2 -> Step execution in progress/Action
  No step running/1(bInterruptStep) -> Merge/1
  Step execution in progress/1(bInterruptStep) -> Merge/2
  Merge/1 -> b_IsStepFinished/1
  st_StepParameters Internal Status/1 -> Step execution in progress/1(stStepParameters)
  b_IsTimerElapsed Internal Status/1 -> Step execution in progress/2(bIsTimeElapsed)
  u16_BatteryVoltage Internal Measure/1 -> Step execution in progress/7(u16BatteryVoltage)
  s32_BeltSpeed Internal Measure/1 -> Step execution in progress/8(s32BeltSpeed)
  b_IsActivePretensioningSituation Project specific/1 -> Step execution in progress/3(bIsNoMoreTensioningSituation)
  u16_Temperature Internal Measure/1 -> Step execution in progress/5(u16Temperature)
  u32_MotorCurrentInmA Internal Measure/1 -> Step execution in progress/4(u32MotorCurrent)
  Logical Operator/1 -> If/1
  Relational Operator/1 -> Logical Operator/2
  Relational Operator1/1 -> Logical Operator/1
  e_StepValidity Internal Status/1 -> Step execution in progress/10(e_StepValidity Internal Status), Relational Operator/2, Relational Operator1/2
  New Step/1 -> Relational Operator1/1
  Step On Going/1 -> Relational Operator/1
  s16_MotorPowerOrder Internal Measure/1 -> Step execution in progress/6(s16MotorPower)
  u16_BeltPayOutFiltered Internal Measure/1 -> Step execution in progress/9(u16BeltPayOutFiltered_mm)

== system LIB_TF_G_12_StepControl/TF_G_12_ControlStepExecution/Extrapolate Next Consign ==
  s32MilliOrderIncrement : Inport  RequirementInfo={} %GIDa_87956398_f0fe_4ec7_92b2_52dfb8590ed8
  s32MilliOrder : Inport  RequirementInfo={} %GIDa_800d2d36_2491_4f91_ba5b_117a54994daf  Port=2
  Add : Sum  RequirementInfo={} %GIDa_6d4f6688_6c83_4d4f_af34_b067c3f62cb4  AccumDataTypeStr=int32  SaturateOnIntegerOverflow=on  mask(TL_Sum){data={'output',{'type','Int32','checkmin',1,'checkmax',1},'date',735951.66801076394}}
      settings: CopyFcn=if exist('tl_reset_reviewflag','file')==2,tl_reset_reviewflag(gcbh);end  DeleteFcn=if exist('delete_tlblock','file')==2,delete_tlblock(gcbh);end  NameChangeFcn=if exist('rename_tlblock','file')==2,rename_tlblock(gcbh);end  OpenFcn=if exist('tl_open_blockdlg','file')==2,tl_open_blockdlg(gcbh);else,open_system(gcbh,'parameter');end
      mask Help: eval(['if exist(''tl_online_help'',''file'') == 2, tl_online_help(''Topic'',''TL_Sum''),else, web([''jar:file:///'',matlabroot,''/help/toolbox/simulink/help.jar!/slref/' lower(get_param(gcbh,'Blocktype')) '.html''], ''-helpbrowser''),end'])
      mask Display: plot([-0.05, 1.05, NaN, -0.05, 1.05],[.01, .01, NaN, .99, .99])
  Add1 : Sum  RequirementInfo={} %GIDa_08d10bdd_dd5e_4709_a416_bde2e3817402  AccumDataTypeStr=int32  OutDataTypeStr=int32  SaturateOnIntegerOverflow=on  mask(TL_Sum){data={'output',{'type','Int32','checkmin',1,'checkmax',1},'date',735951.66801040515}}
      settings: CopyFcn=if exist('tl_reset_reviewflag','file')==2,tl_reset_reviewflag(gcbh);end  DeleteFcn=if exist('delete_tlblock','file')==2,delete_tlblock(gcbh);end  NameChangeFcn=if exist('rename_tlblock','file')==2,rename_tlblock(gcbh);end  OpenFcn=if exist('tl_open_blockdlg','file')==2,tl_open_blockdlg(gcbh);else,open_system(gcbh,'parameter');end
      mask Help: eval(['if exist(''tl_online_help'',''file'') == 2, tl_online_help(''Topic'',''TL_Sum''),else, web([''jar:file:///'',matlabroot,''/help/toolbox/simulink/help.jar!/slref/' lower(get_param(gcbh,'Blocktype')) '.html''], ''-helpbrowser''),end'])
      mask Display: plot([-0.05, 1.05, NaN, -0.05, 1.05],[.01, .01, NaN, .99, .99])
  Constant : Constant  RequirementInfo={} %GIDa_cb53e78c_4b65_404d_bf4d_790a35c25c3d  Value=ddv('Sampling_Freq/KUS_MOTOR_PERIOD')  mask(TL_Constant){data={'output',{'variable','Sampling_Freq/KUS_MOTOR_PERIOD'},'date',735951.66801005788}}
      settings: CopyFcn=if exist('tl_reset_reviewflag','file')==2,tl_reset_reviewflag(gcbh);end  DeleteFcn=if exist('delete_tlblock','file')==2,delete_tlblock(gcbh);end  NameChangeFcn=if exist('rename_tlblock','file')==2,rename_tlblock(gcbh);end  OpenFcn=if exist('tl_open_blockdlg','file')==2,tl_open_blockdlg(gcbh);else,open_system(gcbh,'parameter');end
      mask Help: eval(['if exist(''tl_online_help'',''file'') == 2, tl_online_help(''Topic'',''TL_Constant''),else, web([''jar:file:///'',matlabroot,''/help/toolbox/simulink/help.jar!/slref/' lower(get_param(gcbh,'Blocktype')) '.html''], ''-helpbrowser''),end'])
      mask Display: plot([-0.05, 1.05, NaN, -0.05, 1.05],[.01, .01, NaN, .99, .99])
  Constant1 : Constant  RequirementInfo={} %GIDa_1289af38_90eb_4062_a040_ea0152ace935  Value=ddv('Sampling_Freq/KUS_STEP_SELECTION_PERIOD')  mask(TL_Constant){data={'output',{'variable','Sampling_Freq/KUS_STEP_SELECTION_PERIOD'},'date',735951.66800967592}}
      settings: CopyFcn=if exist('tl_reset_reviewflag','file')==2,tl_reset_reviewflag(gcbh);end  DeleteFcn=if exist('delete_tlblock','file')==2,delete_tlblock(gcbh);end  NameChangeFcn=if exist('rename_tlblock','file')==2,rename_tlblock(gcbh);end  OpenFcn=if exist('tl_open_blockdlg','file')==2,tl_open_blockdlg(gcbh);else,open_system(gcbh,'parameter');end
      mask Help: eval(['if exist(''tl_online_help'',''file'') == 2, tl_online_help(''Topic'',''TL_Constant''),else, web([''jar:file:///'',matlabroot,''/help/toolbox/simulink/help.jar!/slref/' lower(get_param(gcbh,'Blocktype')) '.html''], ''-helpbrowser''),end'])
      mask Display: plot([-0.05, 1.05, NaN, -0.05, 1.05],[.01, .01, NaN, .99, .99])
  Divide : Product  RequirementInfo={} %GIDa_cf020f9f_e377_471f_8cd0_12358ba1b0ec  Inputs=*/  OutDataTypeStr=uint16  mask(TL_Product){data={'output',{'type','UInt8'},'date',735951.66800929396}}
      settings: CopyFcn=if exist('tl_reset_reviewflag','file')==2,tl_reset_reviewflag(gcbh);end  DeleteFcn=if exist('delete_tlblock','file')==2,delete_tlblock(gcbh);end  NameChangeFcn=if exist('rename_tlblock','file')==2,rename_tlblock(gcbh);end  OpenFcn=if exist('tl_open_blockdlg','file')==2,tl_open_blockdlg(gcbh);else,open_system(gcbh,'parameter');end
      mask Help: eval(['if exist(''tl_online_help'',''file'') == 2, tl_online_help(''Topic'',''TL_Product''),else, web([''jar:file:///'',matlabroot,''/help/toolbox/simulink/help.jar!/slref/' lower(get_param(gcbh,'Blocktype')) '.html''], ''-helpbrowser''),end'])
      mask Display: plot([-0.05, 1.05, NaN, -0.05, 1.05],[.01, .01, NaN, .99, .99])
  Product : Product  RequirementInfo={} %GIDa_cdc856fb_af99_424a_9bfd_2217867e9345  OutDataTypeStr=int32  SaturateOnIntegerOverflow=on  RndMeth=Zero  mask(TL_Product){data={'output',{'type','Int32','checkmin',1,'checkmax',1},'date',735951.66800892365}}
      settings: CopyFcn=if exist('tl_reset_reviewflag','file')==2,tl_reset_reviewflag(gcbh);end  DeleteFcn=if exist('delete_tlblock','file')==2,delete_tlblock(gcbh);end  NameChangeFcn=if exist('rename_tlblock','file')==2,rename_tlblock(gcbh);end  OpenFcn=if exist('tl_open_blockdlg','file')==2,tl_open_blockdlg(gcbh);else,open_system(gcbh,'parameter');end
      mask Help: eval(['if exist(''tl_online_help'',''file'') == 2, tl_online_help(''Topic'',''TL_Product''),else, web([''jar:file:///'',matlabroot,''/help/toolbox/simulink/help.jar!/slref/' lower(get_param(gcbh,'Blocktype')) '.html''], ''-helpbrowser''),end'])
      mask Display: plot([-0.05, 1.05, NaN, -0.05, 1.05],[.01, .01, NaN, .99, .99])
  Scope : Scope
      settings: RequirementInfo={} %GIDa_b38e2e82_0511_4374_8d81_424d62d0194d
  SubsystemDetectConsignsChange : Subsystem  RequirementInfo={} %GIDa_7f6dc426_afcd_4aa2_a79a_e2fe2ac13e90  TreatAsAtomicUnit=on
  Switch : Switch  RequirementInfo={} %GIDa_b0436fb6_d5b5_4c63_a622_221b9f50b9ef  Criteria=u2 ~= 0  OutDataTypeStr=int32  mask(TL_Switch){data={'output',{'name','s32EstimatedOrder','inheritscaling',1},'threshold',{'scalar',1},'date',735951.66800672456}}
      settings: CopyFcn=if exist('tl_reset_reviewflag','file')==2,tl_reset_reviewflag(gcbh);end  DeleteFcn=if exist('delete_tlblock','file')==2,delete_tlblock(gcbh);end  NameChangeFcn=if exist('rename_tlblock','file')==2,rename_tlblock(gcbh);end  OpenFcn=if exist('tl_open_blockdlg','file')==2,tl_open_blockdlg(gcbh);else,open_system(gcbh,'parameter');end
      mask Help: eval(['if exist(''tl_online_help'',''file'') == 2, tl_online_help(''Topic'',''TL_Switch''),else, web([''jar:file:///'',matlabroot,''/help/toolbox/simulink/help.jar!/slref/' lower(get_param(gcbh,'Blocktype')) '.html''], ''-helpbrowser''),end'])
      mask Display: plot([-0.05, 1.05, NaN, -0.05, 1.05],[.01, .01, NaN, .99, .99])
  Unit Delay : UnitDelay  RequirementInfo={} %GIDa_95dfe8f0_9f0f_4520_928a_7ba77ed807fa  SampleTime=-1  mask(TL_UnitDelay){data={'output',{'type','Int32'},'state',{'name','s32OldEstimatedOrder','type','Int32'},'date',735951.66800618055}}
      settings: CopyFcn=if exist('tl_reset_reviewflag','file')==2,tl_reset_reviewflag(gcbh);end  DeleteFcn=if exist('delete_tlblock','file')==2,delete_tlblock(gcbh);end  NameChangeFcn=if exist('rename_tlblock','file')==2,rename_tlblock(gcbh);end  OpenFcn=if exist('tl_open_blockdlg','file')==2,tl_open_blockdlg(gcbh);else,open_system(gcbh,'parameter');end
      mask Help: eval(['if exist(''tl_online_help'',''file'') == 2, tl_online_help(''Topic'',''TL_UnitDelay''),else, web([''jar:file:///'',matlabroot,''/help/toolbox/simulink/help.jar!/slref/' lower(get_param(gcbh,'Blocktype')) '.html''], ''-helpbrowser''),end'])
      mask Display: plot([-0.05, 1.05, NaN, -0.05, 1.05],[.01, .01, NaN, .99, .99])
  s32OrderToApply : Outport  RequirementInfo={} %GIDa_d4a9a09e_39a4_46cf_b02e_f6ff3bad6192
  wires:
  s32MilliOrderIncrement/1 -> SubsystemDetectConsignsChange/2(lIncrement), Product/1
  s32MilliOrder/1 -> SubsystemDetectConsignsChange/1(lFirstOrder), Add1/1
  SubsystemDetectConsignsChange/1(bAreConsignsChanged) -> Switch/2
  Switch/1 -> Unit Delay/1, s32OrderToApply/1, Scope/1
  Add/1 -> Switch/3
  Unit Delay/1 -> Add/2
  Add1/1 -> Switch/1
  Constant1/1 -> Divide/1
  Constant/1 -> Divide/2
  Divide/1 -> Product/2
  Product/1 -> Add/1, Add1/2
